simulink model "gm_ldpc_dvbs2_model_v2_fil"  (R2020b)
settings: Solver=FixedStepDiscrete  StartTime=0.0  StopTime=360*135 + 16200  RelTol=1e-3
libraries: simulink x4, hdlsllib x4, hdlmdlgenlib x2, fillib x1
(part 1 of 2)
settings Model: Creator=wardo  LastModifiedBy=EFlores
settings DataIOCC: LimitDataPoints=on  SaveOutput=off  SaveTime=off
settings OptimizationCC: BlockReduction=off  ConditionallyExecuteInputs=off  DefaultParameterBehavior=Inlined  LifeSpan=inf
settings DebuggingCC: AlgebraicLoopMsg=error  InheritedTsInSrcMsg=none  SingleTaskRateTransMsg=error  AllowSymbolicDim=off  StrictBusMsg=ErrorOnBusTreatedAsVector  SFUnexpectedBacktrackingDiag=warning  SFNoUnconditionalDefaultTransitionDiag=warning  SFExecutionAtInitializationDiag=none  ArithmeticOperatorsInVariantConditions=warning
settings HardwareCC: ProdBitPerPointer=32  ProdBitPerSizeT=32  ProdBitPerPtrDiffT=32  ProdLargestAtomicFloat=None  ProdIntDivRoundTo=Undefined  ProdEndianess=Unspecified  ProdWordSize=32  ProdHWDeviceType=ASIC/FPGA->ASIC/FPGA  ProdEqTarget=off
settings SFSimCC: SimUseLocalCustomCode=off  CustomCodeUndefinedFunction=UseInterfaceOnly
settings RTWCC: RTWUseLocalCustomCode=off
settings CodeAppCC: StateflowObjectComments=on
settings GRTTargetCC: TargetLangStandard=C89/C90 (ANSI)
settings ConfigComp: CovScope=ReferencedModels  CovMetricSettings=dw  CovSaveCumulativeToWorkspaceVar=on  CovSaveSingleToWorkspaceVar=on  CovExternalEMLEnable=off  CovSFcnEnable=off

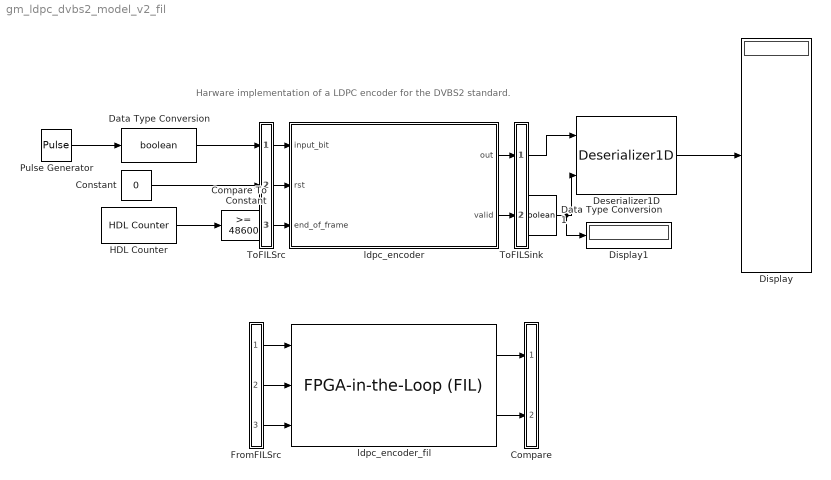
== system gm_ldpc_dvbs2_model_v2_fil ==
  note: Harware implementation of a LDPC encoder for the DVBS2 standard.
  Compare : Subsystem
      mask Display: disp('')
  Compare To Constant : simulink/Logic and Bit Operations/Compare To Constant  relop=>=  const=48600  OutDataTypeStr=boolean
  Constant : Constant  Value=0  OutDataTypeStr=boolean
  Data Type Conversion : DataTypeConversion  OutDataTypeStr=boolean
  Data Type Conversion1 : DataTypeConversion  OutDataTypeStr=boolean
  Deserializer1D : hdlsllib/HDL Operations/Deserializer1D  Ratio=16200  IdleCycles=0  InitialCondition=0  startIn=off  validIn=on  validOut=off  inputDataDimensions=-1  inputSampleTime=-1  inputSignalType=auto
      settings: SourceProductBaseCode=SL
  Display : Display
  Display1 : Display
  FromFILSrc : Subsystem
      mask Display: disp('')
  HDL Counter : hdlsllib/Sources/HDL Counter  CountType=Count limited  CountInit=1  CountStep=1  CountMax=48600  CountFromType=Initial value  CountFrom=1  CountResetPort=off  CountLoadPort=off  CountEnbPort=off  CountDirPort=off  CountDataType=Unsigned  CountWordLen=16  CountFracLen=0  CountSampTime=1
  Pulse Generator : DiscretePulseGenerator  PulseType=Time based  PulseWidth=50
  ToFILSink : Subsystem
      mask Display: disp('')
  ToFILSrc : Subsystem
      mask Display: disp('')
  ldpc_encoder : Subsystem
  ldpc_encoder_fil : fillib/FPGA-in-the-Loop (FIL)  ForceInterfaceUpdate=0.90579
      settings: SourceProductBaseCode=ES,HD
  wires:
  Pulse Generator/1 -> Data Type Conversion/1
  HDL Counter/1 -> Compare To Constant/1
  Deserializer1D/1 -> Display/1
  Data Type Conversion1/1 -> Deserializer1D/2, Display1/1
  ToFILSrc/1(out1) -> ldpc_encoder/1(input_bit)
  ToFILSrc/2(out2) -> ldpc_encoder/2(rst)
  ToFILSrc/3(out3) -> ldpc_encoder/3(end_of_frame)
  ldpc_encoder/1(out) -> ToFILSink/1(in1)
  ldpc_encoder/2(valid) -> ToFILSink/2(in2)
  Data Type Conversion/1 -> ToFILSrc/1(in1)
  Constant/1 -> ToFILSrc/2(in2)
  Compare To Constant/1 -> ToFILSrc/3(in3)
  ToFILSink/1(out1) -> Deserializer1D/1
  ToFILSink/2(out2) -> Data Type Conversion1/1
  FromFILSrc/1(out1) -> ldpc_encoder_fil/1
  FromFILSrc/2(out2) -> ldpc_encoder_fil/2
  FromFILSrc/3(out3) -> ldpc_encoder_fil/3
  ldpc_encoder_fil/1 -> Compare/1(in1)
  ldpc_encoder_fil/2 -> Compare/2(in2)

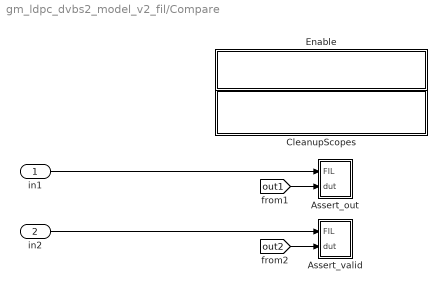
== system gm_ldpc_dvbs2_model_v2_fil/Compare ==
  in1 : Inport
  in2 : Inport  Port=2
  Assert_out : Subsystem
  Assert_valid : Subsystem
  CleanupScopes : Subsystem
      settings: OpenFcn=|
      | blkName = gcb; %self block
      | idx = regexp(blkName, '/CleanupScopes$', 'once');
      | blkParent = blkName(1:idx-1);
      | blks=find_system(blkParent, 'LookUnderMasks', 'all','blocktype', 'Scope');
      | for itr = 1:length(blks)
      | 	 hScopeCfg = get_param(blks{itr},'ScopeConfiguration');
      | 	 hScopeCfg.Visible = ~ hScopeCfg.Visible;
      | end
      | drawnow;
      mask Display: fprintf(message('hdlcoder:cosim:vnl_dblclick').getString());
  Enable : Subsystem
      settings: OpenFcn=|
      | blkName = gcb;
      | idx = regexp(blkName, '/Enable$', 'once');
      | blkParent = blkName(1:idx-1);
      | blks=find_system(blkParent, 'LookUnderMasks', 'all','blocktype', 'Assertion');
      | e = get_param(blks{1}, 'Enabled');
      | if strcmp(e, 'on'), f= 'off';, else, f = 'on';, end
      | for ii=1:length(blks), set_param(blks{ii}, 'Enabled', f);, end
      | set_param(gcb, 'MaskDisplay',['fprintf(message(''hdlcoder:cosim:vnl_dblclick_assertions'',','''',upper(e),'''',').getString())']);
      mask Display: fprintf(message('hdlcoder:cosim:vnl_dblclick_assertions','OFF').getString());
  wires:
  in1/1 -> Assert_out/1(FIL)
  [out1] -> Assert_out/2(dut)
  in2/1 -> Assert_valid/1(FIL)
  [out2] -> Assert_valid/2(dut)

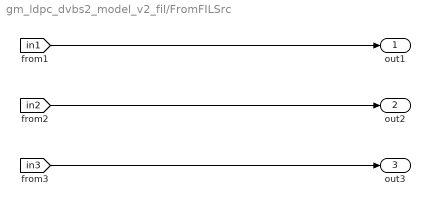
== system gm_ldpc_dvbs2_model_v2_fil/FromFILSrc ==
  out1 : Outport
  out2 : Outport  Port=2
  out3 : Outport  Port=3
  wires:
  [in1] -> out1/1
  [in2] -> out2/1
  [in3] -> out3/1

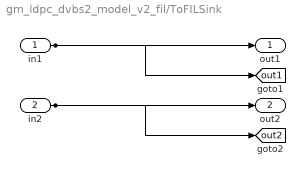
== system gm_ldpc_dvbs2_model_v2_fil/ToFILSink ==
  in1 : Inport
  in2 : Inport  Port=2
  out1 : Outport
  out2 : Outport  Port=2
  tag scope: out1=global, out2=global
  wires:
  in1/1 -> out1/1, [out1]
  in2/1 -> out2/1, [out2]

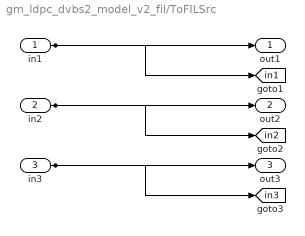
== system gm_ldpc_dvbs2_model_v2_fil/ToFILSrc ==
  in1 : Inport
  in2 : Inport  Port=2
  in3 : Inport  Port=3
  out1 : Outport
  out2 : Outport  Port=2
  out3 : Outport  Port=3
  tag scope: in1=global, in2=global, in3=global
  wires:
  in1/1 -> out1/1, [in1]
  in2/1 -> out2/1, [in2]
  in3/1 -> out3/1, [in3]

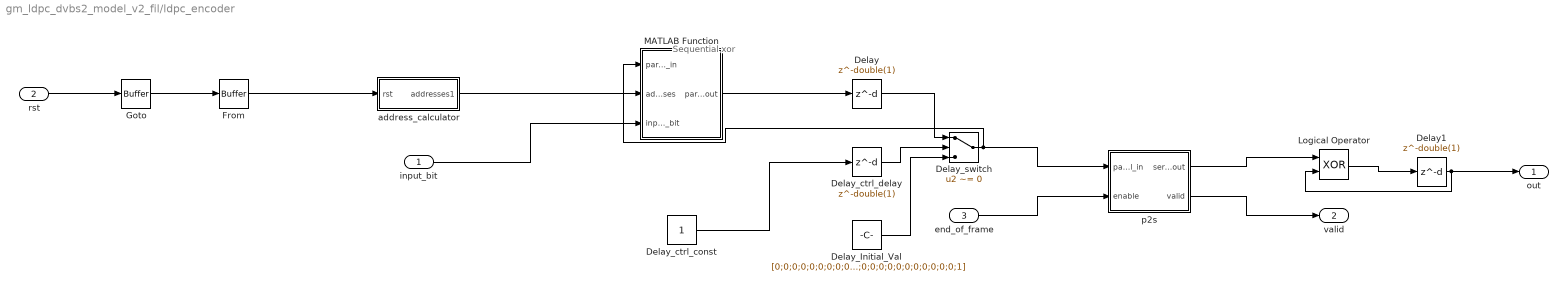
== system gm_ldpc_dvbs2_model_v2_fil/ldpc_encoder ==
  note: Sequential xor
  input_bit : Inport  OutDataTypeStr=boolean  PortDimensions=1  SampleTime=1
  rst : Inport  Port=2  OutDataTypeStr=boolean  PortDimensions=1
  end_of_frame : Inport  Port=3  OutDataTypeStr=boolean  PortDimensions=1  SampleTime=1
  Delay : Delay  DelayLength=double(1)  InitialCondition=0  SampleTime=1
  Delay1 : Delay  DelayLength=double(1)  InitialCondition=0  SampleTime=1
  Delay_Initial_Val : Constant  Value=[0;0;0;0;0;0;0;0;0;0;0;0;0;0;0;0;0;0;0;0;0;0;0;0;0;0;0;0;0;0;0;0;0;0;0;0;0;0;0;0;0;0;0;0;0;0;0;0;0;0;0;0;0;0;0;0;0;0;0;0;0;0;0;0;0;0;0;0;0;0;0;0;0;0;0;0;0;0;0;0;0;0;0;0;0;0;0;0;0;0;0;0;0;0;0;0;0;0;0;0;0;0;0;0;0;0;0;0;0;0;0;0;0;0;0;0;0;0;0;0;0;0;0;0;0;0;0;0;0;0;0;0;0;0;0;0;0;0;0;0;0;0;0;0;0;0;0;0;0;0;0;0;0;0;0;0;0;0;0;0;0;0;0;0;0;0;0;0;0;0;0;0;0;0;0;0;0;0;0;0;0;0;0;0;0;0;0;0;0;0;0;0;0;0;0;0;0;0;0;0;0;0;0;0;0;0;0;0;0;0;0;0;0;0;0;0;0;0;0;0;0;0;0;0;0;0;0;0;0;0;0;0;0;0;0;0;0;0;0;0;0;0;0;0;0;0;0;0;0;0;0;0;0;0;0;0;0;0;0;0;0;0;0;0;0;0;0;0;0;0;0;0;0;0;0;0;0;0;0;0;0;0;0;0;0;0;0;0;0;0;0;0;0;0;0;0;0;0;0;0;0;0;0;0;0;0;0;0;0;0;0;0;0;0;0;0;0;0;0;0;0;0;0;0;0;0;0;0;0;0;0;0;0;0;0;0;0;0;0;0;0;0;0;0;0;0;0;0;0;0;0;0;0;0;0;0;0;0;0;0;0;0;0;0;0;0;0;0;0;0;0;0;0;0;0;0;0;0;0;0;0;0;0;0;0;0;0;0;0;0;0;0;0;0;0;0;0;0;0;0;0;0;0;0;0;0;0;0;0;0;0;0;0;0;0;0;0;0;0;0;0;0;0;0;0;0;0;0;0;0;0;0;0;0;0;0;0;0;0;0;0;0;0;0;0;0;0;0;0;0;0;0;0;0;0;0;0;0;0;0;0;0;0;0;0;0;0;0;0;0;0;0;0;0;0;0;0;0;0;0;0;0;0;0;0;0;0;0;0;0;0;0;0;0;0;0;0;0;0;0;0;0;0;0;0;0;0;0;0;0;0;0;0;0;0;0;0;0;0;0;0;0;0;0;0;0;0;0;0;0;0;0;0;0;0;0;0;0;0;0;0;0;0;0;0;0;0;0;0;0;0;0;0;0;0;0;0;0;0;0;0;0;0;0;0;0;0;0;0;0;0;0;0;0;0;0;0;0;0;0;0;0;0;0;0;0;0;0;0;0;0;0;0;0;0;0;0;0;0;0;0;0;0;0;0;0;0;0;0;0;0;0;0;0;0;0;0;0;0;0;0;0;0;0;0;0;0;0;0;0;0;0;0;0;0;0;0;0;0;0;0;0;0;0;0;0;0;0;0;0;0;0;0;0;0;0;0;0;0;0;0;0;0;0;0;0;0;0;0;0;0;0;0;0;0;0;0;0;0;0;0;0;0;0;0;0;0;0;0;0;0;0;0;0;0;0;0;0;0;0;0;0;0;0;0;0;0;0;0;0;0;0;0;0;0;0;0;0;0;0;0;0;0;0;0;0;0;0;0;0;0;0;0;0;0;0;0;0;0;0;0;0;0;0;0;0;0;0;0;0;0;0;0;0;0;0;0;0;0;0;0;0;0;0;0;0;0;0;0;0;0;0;0;0;0;0;0;0;0;0;0;0;0;0;0;0;0;0;0;0;0;0;0;0;0;0;0;0;0;0;0;0;0;0;0;0;0;0;0;0;0;0;0;0;0;0;0;0;0;0;0;0;0;0;0;0;0;0;0;0;0;0;0;0;0;0;0;0;0;0;0;0;0;0;0;0;0;0;0;0;0;0;0;0;0;0;0;0;0;0;0;0;0;0;0;0;0;0;0;0;0;0;0;0;0;0;0;0;0;0;0;0;0;0;0;0;0;0;0;0;0;0;0;0;0;0;0;0;0;0;0;0;0;0;0;0;0;0;0;0;0;0;0;0;0;0;0;0;0;0;0;0;0;0;0;0;0;0;0;0;0;0;0;0;0;0;0;0;0;0;0;0;0;0;0;0;0;0;0;0;0;0;0;0;0;0;0;0;0;0;0;0;0;0;0;0;0;0;0;0;0;0;0;0;0;0;0;0;0;0;0;0;0;0;0;0;0;0;0;0;0;0;0;0;0;0;0;0;0;0;0;0;0;0;0;0;0;0;0;0;0;0;0;0;0;0;0;0;0;0;0;0;0;0;0;0;0;0;0;0;0;0;0;0;0;0;0;0;0;0;0;0;0;0;0;0;0;0;0;0;0;0;0;0;0;0;0;0;0;0;0;0;0;0;0;0;0;0;0;0;0;0;0;0;0;0;0;0;0;0;0;0;0;0;0;0;0;0;0;0;0;0;0;0;0;0;0;0;0;0;0;0;0;0;0;0;0;0;0;0;0;0;0;0;0;0;0;0;0;0;0;0;0;0;0;0;0;0;0;0;0;0;0;0;0;0;0;0;0;0;0;0;0;0;0;0;0;0;0;0;0;0;0;0;0;0;0;0;0;0;0;0;0;0;0;0;0;0;0;0;0;0;0;0;0;0;0;0;0;0;0;0;0;0;0;0;0;0;0;0;0;0;0;0;0;0;0;0;0;0;0;0;0;0;0;0;0;0;0;0;0;0;0;0;0;0;0;0;0;0;0;0;0;0;0;0;0;0;0;0;0;0;0;0;0;0;0;0;0;0;0;0;0;0;0;0;0;0;0;0;0;0;0;0;0;0;0;0;0;0;0;0;0;0;0;0;0;0;0;0;0;0;0;0;0;0;0;0;0;0;0;0;0;0;0;0;0;0;0;0;0;0;0;0;0;0;0;0;0;0;0;0;0;0;0;0;0;0;0;0;0;0;0;0;0;0;0;0;0;0;0;0;0;0;0;0;0;0;0;0;0;0;0;0;0;0;0;0;0;0;0;0;0;0;0;0;0;0;0;0;0;0;0;0;0;0;0;0;0;0;0;0;0;0;0;0;0;0;0;0;0;0;0;0;0;0;0;0;0;0;0;0;0;0;0;0;0;0;0;0;0;0;0;0;0;0;0;0;0;0;0;0;0;0;0;0;0;0;0;0;0;0;0;0;0;0;0;0;0;0;0;0;0;0;0;0;0;0;0;0;0;0;0;0;0;0;0;0;0;0;0;0;0;0;0;0;0;0;0;0;0;0;0;0;0;0;0;0;0;0;0;0;0;0;0;0;0;0;0;0;0;0;0;0;0;0;0;0;0;0;0;0;0;0;0;0;0;0;0;0;0;0;0;0;0;0;0;0;0;0;0;0;0;0;0;0;0;0;0;0;0;0;0;0;0;0;0;0;0;0;0;0;0;0;0;0;0;0;0;0;0;0;0;0;0;0;0;0;0;0;0;0;0;0;0;0;0;0;0;0;0;0;0;0;0;0;0;0;0;0;0;0;0;0;0;0;0;0;0;0;0;0;0;0;0;0;0;0;0;0;0;0;0;0;0;0;0;0;0;0;0;0;0;0;0;0;0;0;0;0;0;0;0;0;0;0;0;0;0;0;0;0;0;0;0;0;0;0;0;0;0;0;0;0;0;0;0;0;0;0;0;0;0;0;0;0;0;0;0;0;0;0;0;0;0;0;0;0;0;0;0;0;0;0;0;0;0;0;0;0;0;0;0;0;0;0;0;0;0;0;0;0;0;0;0;0;0;0;0;0;0;0;0;0;0;0;0;0;0;0;0;0;0;0;0;0;0;0;0;0;0;0;0;0;0;0;0;0;0;0;0;0;0;0;0;0;0;0;0;0;0;0;0;0;0;0;0;0;0;0;0;0;0;0;0;0;0;0;0;0;0;0;0;0;0;0;0;0;0;0;0;0;0;0;0;0;0;0;0;0;0;0;0;0;0;0;0;0;0;0;0;0;0;0;0;0;0;0;0;0;0;0;0;0;0;0;0;0;0;0;0;0;0;0;0;0;0;0;0;0;0;0;0;0;0;0;0;0;0;0;0;0;0;0;0;0;0;0;0;0;0;0;0;0;0;0;0;0;0;0;0;0;0;0;0;0;0;0;0;0;0;0;0;0;0;0;0;0;0;0;0;0;0;0;0;0;0;0;0;0;0;0;0;0;0;0;0;0;0;0;0;0;0;0;0;0;0;0;0;0;0;0;0;0;0;0;0;0;0;0;0;0;0;0;0;0;0;0;0;0;0;0;0;0;0;0;0;0;0;0;0;0;0;0;0;0;0;0;0;0;0;0;0;0;0;0;0;0;0;0;0;0;0;0;0;0;0;0;0;0;0;0;0;0;0;0;0;0;0;0;0;0;0;0;0;0;0;0;0;0;0;0;0;0;0;0;0;0;0;0;0;0;0;0;0;0;0;0;0;0;0;0;0;0;0;0;0;0;0;0;0;0;0;0;0;0;0;0;0 ...(+28404 chars)]  OutDataTypeStr=fixdt(0, 1, 0)  SampleTime=1
  Delay_ctrl_const : Constant  OutDataTypeStr=boolean  SampleTime=1
  Delay_ctrl_delay : Delay  DelayLength=double(1)  InitialCondition=0  SampleTime=1
  Delay_switch : Switch  Criteria=u2 ~= 0  Threshold=double(0)  OutDataTypeStr=fixdt(0, 1, 0)  SampleTime=1
  From : hdlmdlgenlib/Buffer
      settings: SourceProductBaseCode=SL
  Goto : hdlmdlgenlib/Buffer
      settings: SourceProductBaseCode=SL
  Logical Operator : Logic  Operator=XOR  AllPortsSameDT=off  OutDataTypeStr=fixdt(0, 1, 0)  SampleTime=1
  MATLAB Function : Subsystem
  address_calculator : Subsystem
  p2s : Subsystem
  out : Outport  VectorParamsAs1DForOutWhenUnconnected=off
  valid : Outport  Port=2  VectorParamsAs1DForOutWhenUnconnected=off
  wires:
  Delay_ctrl_delay/1 -> Delay_switch/2
  Delay_ctrl_const/1 -> Delay_ctrl_delay/1
  Delay_Initial_Val/1 -> Delay_switch/3
  Delay/1 -> Delay_switch/1
  Goto/1 -> From/1
  p2s/2(valid) -> valid/1
  p2s/1(serial_out) -> Logical Operator/1
  address_calculator/1(addresses1) -> MATLAB Function/2(addresses)
  MATLAB Function/1(parity_out) -> Delay/1
  Logical Operator/1 -> Delay1/1
  From/1 -> address_calculator/1(rst)
  Delay1/1 -> out/1, Logical Operator/2
  Delay_switch/1 -> MATLAB Function/1(parity_in), p2s/1(parallel_in)
  end_of_frame/1 -> p2s/2(enable)
  rst/1 -> Goto/1
  input_bit/1 -> MATLAB Function/3(input_bit)

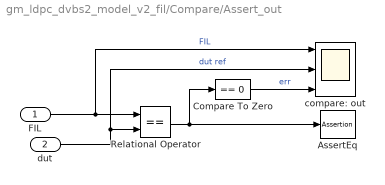
== system gm_ldpc_dvbs2_model_v2_fil/Compare/Assert_out ==
  FIL : Inport
  dut : Inport  Port=2
  AssertEq : Assertion  StopWhenAssertionFail=off
  Compare To Zero : simulink/Logic and Bit Operations/Compare To Zero  relop===  OutDataTypeStr=boolean
  Relational Operator : RelationalOperator  Operator===  OutDataTypeStr=boolean  RndMeth=Nearest
  compare: out : Scope  NumInputPorts=3
  wires:
  Compare To Zero/1 -> compare: out/3  "err"
  Relational Operator/1 -> Compare To Zero/1, AssertEq/1
  FIL/1 -> compare: out/1, Relational Operator/1  "FIL"
  dut/1 -> compare: out/2, Relational Operator/2  "dut ref"

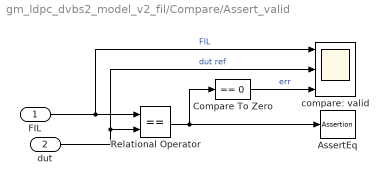
== system gm_ldpc_dvbs2_model_v2_fil/Compare/Assert_valid ==
  FIL : Inport
  dut : Inport  Port=2
  AssertEq : Assertion  StopWhenAssertionFail=off
  Compare To Zero : simulink/Logic and Bit Operations/Compare To Zero  relop===  OutDataTypeStr=boolean
  Relational Operator : RelationalOperator  Operator===  OutDataTypeStr=boolean  RndMeth=Nearest
  compare: valid : Scope  NumInputPorts=3
  wires:
  Compare To Zero/1 -> compare: valid/3  "err"
  Relational Operator/1 -> Compare To Zero/1, AssertEq/1
  FIL/1 -> compare: valid/1, Relational Operator/1  "FIL"
  dut/1 -> compare: valid/2, Relational Operator/2  "dut ref"

== system gm_ldpc_dvbs2_model_v2_fil/Compare/CleanupScopes ==

== system gm_ldpc_dvbs2_model_v2_fil/Compare/Enable ==

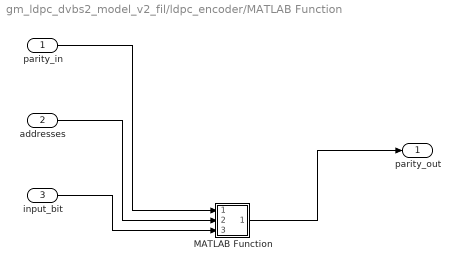
== system gm_ldpc_dvbs2_model_v2_fil/ldpc_encoder/MATLAB Function ==
  parity_in : Inport  OutDataTypeStr=fixdt(0, 1, 0)  PortDimensions=[16201]  SampleTime=1
  addresses : Inport  Port=2  OutDataTypeStr=uint16  PortDimensions=[1 12]  SampleTime=1
  input_bit : Inport  Port=3  OutDataTypeStr=boolean  PortDimensions=1  SampleTime=1
  MATLAB Function : MATLAB Function  TreatAsAtomicUnit=on
  parity_out : Outport  VectorParamsAs1DForOutWhenUnconnected=off
  wires:
  MATLAB Function/1(parity_out) -> parity_out/1
  input_bit/1 -> MATLAB Function/3(input_bit)
  addresses/1 -> MATLAB Function/2(addresses)
  parity_in/1 -> MATLAB Function/1(parity_in)

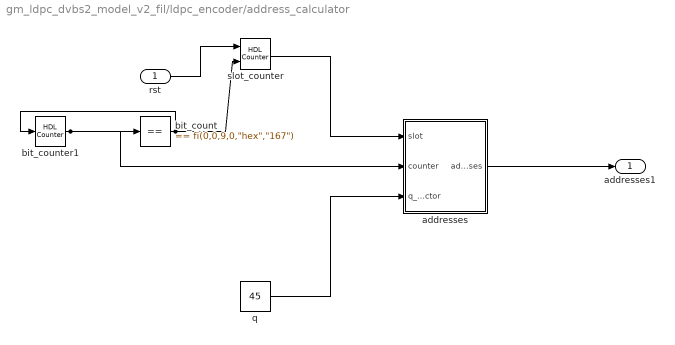
== system gm_ldpc_dvbs2_model_v2_fil/ldpc_encoder/address_calculator ==
  rst : Inport  OutDataTypeStr=boolean  PortDimensions=1
  addresses : Subsystem
  bit_count : simulink/Logic and Bit Operations/Compare To Constant  relop===  const="fi(0,0,9,0,\"hex\",\"167\")"  OutDataTypeStr=boolean
  bit_counter1 : hdlsllib/Sources/HDL Counter  CountType=Count limited  CountInit=double(0)  CountStep=double(1)  CountMax=double(359)  CountFromType=Initial value  CountFrom=double(0)  CountResetPort=on  CountLoadPort=off  CountEnbPort=off  CountDirPort=off  CountDataType=Unsigned  CountWordLen=9  CountFracLen=0  CountSampTime=1
  q : Constant  Value=45  OutDataTypeStr=uint8  SampleTime=1
  slot_counter : hdlsllib/Sources/HDL Counter  CountType=Count limited  CountInit=double(1)  CountStep=double(1)  CountMax=double(135)  CountFromType=Initial value  CountFrom=double(1)  CountResetPort=on  CountLoadPort=off  CountEnbPort=on  CountDirPort=off  CountDataType=Unsigned  CountWordLen=8  CountFracLen=0  CountSampTime=1
  addresses1 : Outport
  wires:
  slot_counter/1 -> addresses/1(slot)
  q/1 -> addresses/3(q_factor)
  bit_counter1/1 -> addresses/2(counter), bit_count/1
  bit_count/1 -> bit_counter1/1, slot_counter/2
  addresses/1(addresses) -> addresses1/1
  rst/1 -> slot_counter/1

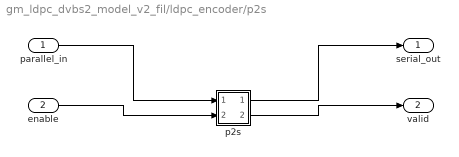
== system gm_ldpc_dvbs2_model_v2_fil/ldpc_encoder/p2s ==
  parallel_in : Inport  OutDataTypeStr=fixdt(0, 1, 0)  PortDimensions=[16201]  SampleTime=1
  enable : Inport  Port=2  OutDataTypeStr=boolean  PortDimensions=1  SampleTime=1
  p2s : MATLAB Function  TreatAsAtomicUnit=on  mask{input_length=16200}
  serial_out : Outport  VectorParamsAs1DForOutWhenUnconnected=off
  valid : Outport  Port=2
  wires:
  p2s/2(valid) -> valid/1
  p2s/1(serial_out) -> serial_out/1
  enable/1 -> p2s/2(enable)
  parallel_in/1 -> p2s/1(parallel_in)
